simulink model "IEEE5BusSystemModel"  (R2017a)
settings: Solver=VariableStepAuto  StartTime=0.0  StopTime=1  MaxStep=1e-4  RelTol=1e-3  EnableMultiTasking=on
libraries: powerlib x45
settings Model: Creator=Rodney Tan  LastModifiedBy=HP
settings OptimizationCC: LifeSpan=inf
settings DebuggingCC: SFUnexpectedBacktrackingDiag=warning  SFNoUnconditionalDefaultTransitionDiag=warning  SFExecutionAtInitializationDiag=none
settings GRTTargetCC: TargetLangStandard=C89/C90 (ANSI)  GeneratePreprocessorConditionals=Disable all
settings ConfigComp: CovMetricSettings=dw  CovHtmlReporting=on  CovSaveCumulativeToWorkspaceVar=on  CovSaveSingleToWorkspaceVar=on  CovExternalEMLEnable=off

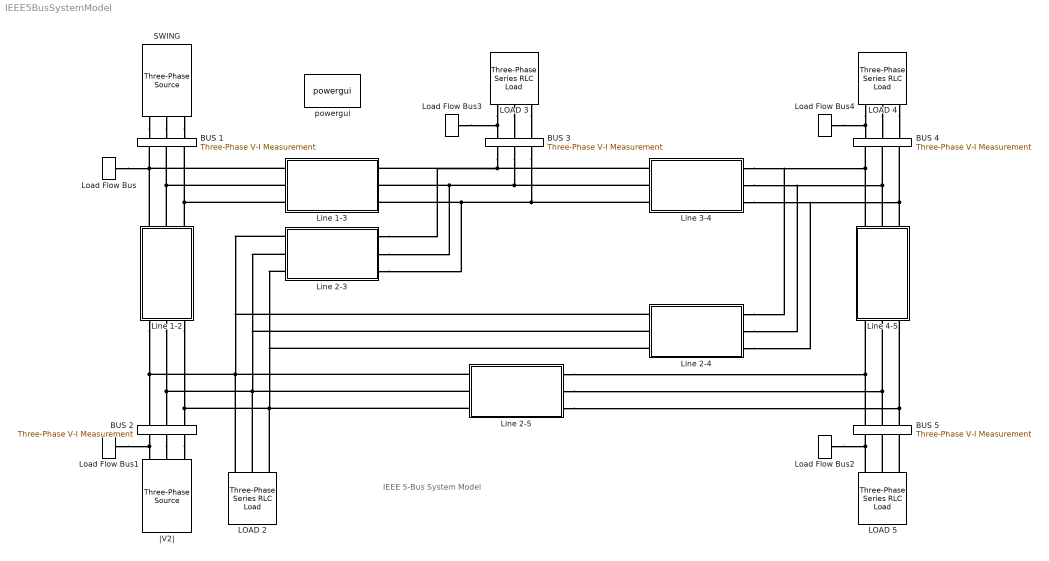
== system IEEE5BusSystemModel ==
  note: IEEE 5-Bus System Model
  BUS {1..5} (5 alike) : powerlib/Measurements/Three-Phase V-I Measurement  VoltageMeasurement=no  SetLabelV=off  LabelV=Vabc  Vpu=off  VpuLL=off  CurrentMeasurement=no  SetLabelI=off  LabelI=Iabc  Ipu=off  Pbase=100e6  Vbase=500e3  OutputType=Complex  PhasorSimulation=off  PSBequivalent=0
  LOAD 2 : powerlib/Elements/Three-Phase Series RLC Load  LConnTagsString=A|B|C  Configuration=Y (grounded)  NominalVoltage=10000  Vabc=[1e3 1e3 1e3]  Vabcp=[1e3 1e3 1e3]  NominalFrequency=60  UnbalancedPower=off  ActivePower=20e6  InductivePower=10e6  CapacitivePower=0  Pabc=[10e3 9e3 11e3]  QLabc=[100 90 110]  QCabc=[100 90 110]  Pabcp=[10e3 9e3 11e3]  QLabcp=[100 90 110]  QCabcp=[100 90 110]  Measurements=None  LoadType=constant PQ
  LOAD 3 : powerlib/Elements/Three-Phase Series RLC Load  LConnTagsString=A|B|C  Configuration=Y (grounded)  NominalVoltage=10000  Vabc=[1e3 1e3 1e3]  Vabcp=[1e3 1e3 1e3]  NominalFrequency=60  UnbalancedPower=off  ActivePower=45e6  InductivePower=15e6  CapacitivePower=0  Pabc=[10e3 9e3 11e3]  QLabc=[100 90 110]  QCabc=[100 90 110]  Pabcp=[10e3 9e3 11e3]  QLabcp=[100 90 110]  QCabcp=[100 90 110]  Measurements=None  LoadType=constant PQ
  LOAD 4 : powerlib/Elements/Three-Phase Series RLC Load  LConnTagsString=A|B|C  Configuration=Y (grounded)  NominalVoltage=(10000)  Vabc=[1e3 1e3 1e3]  Vabcp=[1e3 1e3 1e3]  NominalFrequency=60  UnbalancedPower=off  ActivePower=40e6  InductivePower=5e6  CapacitivePower=0  Pabc=[10e3 9e3 11e3]  QLabc=[100 90 110]  QCabc=[100 90 110]  Pabcp=[10e3 9e3 11e3]  QLabcp=[100 90 110]  QCabcp=[100 90 110]  Measurements=None  LoadType=constant PQ
  LOAD 5 : powerlib/Elements/Three-Phase Series RLC Load  LConnTagsString=A|B|C  Configuration=Y (grounded)  NominalVoltage=10000  Vabc=[1e3 1e3 1e3]  Vabcp=[1e3 1e3 1e3]  NominalFrequency=60  UnbalancedPower=off  ActivePower=60e6  InductivePower=10e6  CapacitivePower=0  Pabc=[10e3 9e3 11e3]  QLabc=[100 90 110]  QCabc=[100 90 110]  Pabcp=[10e3 9e3 11e3]  QLabcp=[100 90 110]  QCabcp=[100 90 110]  Measurements=None  LoadType=constant PQ
  Line 1-2 : Subsystem  mask{F=60, R=0.02, xL=0.06, B=0.03}
      mask prompts: F "Line Frequency (Hz)"; R "Line Resistance (pu)"; xL "Line Inductance (pu)"; B "Line Susceptance (pu)"
      mask Display:
      | disp('Line');
      | port_label('lconn',1,'A');
      | port_label('lconn',2,'B');
      | port_label('lconn',3,'C');
      | port_label('rconn',1,'a');
      | port_label('rconn',2,'b');
      | port_label('rconn',3,'c');
  Line 1-3 : Subsystem  mask{F=60, R=0.08, xL=0.24, B=0.025}
      mask prompts: F "Line Frequency (Hz)"; R "Line Resistance (pu)"; xL "Line Inductance (pu)"; B "Line Susceptance (pu)"
      mask Display:
      | disp('Line');
      | port_label('lconn',1,'A');
      | port_label('lconn',2,'B');
      | port_label('lconn',3,'C');
      | port_label('rconn',1,'a');
      | port_label('rconn',2,'b');
      | port_label('rconn',3,'c');
  Line 2-3 : Subsystem  mask{F=60, R=0.06, xL=0.18, B=0.02}
      mask prompts: F "Line Frequency (Hz)"; R "Line Resistance (pu)"; xL "Line Inductance (pu)"; B "Line Susceptance (pu)"
      mask Display:
      | disp('Line');
      | port_label('lconn',1,'A');
      | port_label('lconn',2,'B');
      | port_label('lconn',3,'C');
      | port_label('rconn',1,'a');
      | port_label('rconn',2,'b');
      | port_label('rconn',3,'c');
  Line 2-4 : Subsystem  mask{F=60, R=0.06, xL=0.18, B=0.02}
      mask prompts: F "Line Frequency (Hz)"; R "Line Resistance (pu)"; xL "Line Inductance (pu)"; B "Line Susceptance (pu)"
      mask Display:
      | disp('Line');
      | port_label('lconn',1,'A');
      | port_label('lconn',2,'B');
      | port_label('lconn',3,'C');
      | port_label('rconn',1,'a');
      | port_label('rconn',2,'b');
      | port_label('rconn',3,'c');
  Line 2-5 : Subsystem  mask{F=60, R=0.04, xL=0.12, B=0.015}
      mask prompts: F "Line Frequency (Hz)"; R "Line Resistance (pu)"; xL "Line Inductance (pu)"; B "Line Susceptance (pu)"
      mask Display:
      | disp('Line');
      | port_label('lconn',1,'A');
      | port_label('lconn',2,'B');
      | port_label('lconn',3,'C');
      | port_label('rconn',1,'a');
      | port_label('rconn',2,'b');
      | port_label('rconn',3,'c');
  Line 3-4 : Subsystem  mask{F=60, R=0.01, xL=0.03, B=0.01}
      mask prompts: F "Line Frequency (Hz)"; R "Line Resistance (pu)"; xL "Line Inductance (pu)"; B "Line Susceptance (pu)"
      mask Display:
      | disp('Line');
      | port_label('lconn',1,'A');
      | port_label('lconn',2,'B');
      | port_label('lconn',3,'C');
      | port_label('rconn',1,'a');
      | port_label('rconn',2,'b');
      | port_label('rconn',3,'c');
  Line 4-5 : Subsystem  mask{F=60, R=0.08, xL=0.24, B=0.025}
      mask prompts: F "Line Frequency (Hz)"; R "Line Resistance (pu)"; xL "Line Inductance (pu)"; B "Line Susceptance (pu)"
      mask Display:
      | disp('Line');
      | port_label('lconn',1,'A');
      | port_label('lconn',2,'B');
      | port_label('lconn',3,'C');
      | port_label('rconn',1,'a');
      | port_label('rconn',2,'b');
      | port_label('rconn',3,'c');
  Load Flow Bus : powerlib/Measurements/Load Flow Bus  LConnTagsString=a  Phases=single  Connectors=on one side  ID=BUS_1  Vbase=10e3  Vref=1.06  Vangle=0  VLF=1.06  VLFb=1  VLFc=1  angleLF=0  angleLFb=0  angleLFc=0
      settings: SourceProductName=Simscape Power Systems
  Load Flow Bus1 : powerlib/Measurements/Load Flow Bus  LConnTagsString=a  Phases=single  Connectors=on one side  ID=BUS_2  Vbase=10e3  Vref=1  Vangle=0  VLF=1.047  VLFb=1  VLFc=1  angleLF=-2.806  angleLFb=0  angleLFc=0
      settings: SourceProductName=Simscape Power Systems
  Load Flow Bus2 : powerlib/Measurements/Load Flow Bus  LConnTagsString=a  Phases=single  Connectors=on one side  ID=BUS_5  Vbase=10e3  Vref=1  Vangle=0  VLF=1.018  VLFb=1  VLFc=1  angleLF=-6.15  angleLFb=0  angleLFc=0
      settings: SourceProductName=Simscape Power Systems
  Load Flow Bus3 : powerlib/Measurements/Load Flow Bus  LConnTagsString=a  Phases=single  Connectors=on one side  ID=BUS_3  Vbase=10e3  Vref=1  Vangle=0  VLF=1.024  VLFb=1  VLFc=1  angleLF=-4.997  angleLFb=0  angleLFc=0
      settings: SourceProductName=Simscape Power Systems
  Load Flow Bus4 : powerlib/Measurements/Load Flow Bus  LConnTagsString=a  Phases=single  Connectors=on one side  ID=BUS_4  Vbase=10e3  Vref=1  Vangle=0  VLF=1.024  VLFb=1  VLFc=1  angleLF=-5.329  angleLFb=0  angleLFc=0
      settings: SourceProductName=Simscape Power Systems
  SWING : powerlib/Electrical Sources/Three-Phase Source  InternalConnection=Yg  VoltagePhases=off  Voltage=(10000)*1.06  PhaseAngle=0  Voltage_phases=[25e3 25e3 25e3]/sqrt(3)  PhaseAngles_phases=[0 -120 +120]  Frequency=60  NonIdealSource=off  SpecifyImpedance=off  Resistance=0.8929  Inductance=16.58e-3  ShortCircuitLevel=100e6  BaseVoltage=25e3  XRratio=7  BusType=swing  Pref=10e3  Qref=0  Prefabc=[10e3, 10e3, 10e3]  Qrefabc=[0, 0, 0]  Qmin=0  Qmax=0
  powergui : powerlib/powergui  Priority=1  SimulationMode=Continuous  SampleTime=50e-6  frequency=60  Iterations=50  frequencyindice=60  Pbase=100e6  ErrMax=0.0001  UnitsV=kV  UnitsW=MW  buscounter=0  FunctionMessages=off  echomessages=off  EnableUseOfTLC=off  CurrentSourceSwitches=off  DisableSnubberDevices=off  DisableRonSwitches=off  DisableVfSwitches=off  DisplayEquations=off  SolverType=Tustin/Backward Euler (TBE)  Interpol=off  ExternalGateDelay=off  methode=off  Ts=100  x0status=blocks  SPID=on  SwTol=0  HookPort=off  RestoreLinks=warning  ResistiveCurrentMeasurement=off  Frange=[0:2:500]  Ylog=off  Xlog=on  ShowGrid=off  save=off  variable=ZData  structure=0  ZoomFFT=off  StartTime=0.0  cycles=1  DisplayStyle=1  fundamental=60  FreqAxis=off  MaxFrequency=1000  frequencyindicesteady=1  RmsSteady=1  display=off
  |V2| : powerlib/Electrical Sources/Three-Phase Source  InternalConnection=Yg  VoltagePhases=off  Voltage=10000  PhaseAngle=0  Voltage_phases=[25e3 25e3 25e3]/sqrt(3)  PhaseAngles_phases=[0 -120 +120]  Frequency=60  NonIdealSource=off  SpecifyImpedance=off  Resistance=0.8929  Inductance=16.58e-3  ShortCircuitLevel=100e6  BaseVoltage=25e3  XRratio=7  BusType=PV  Pref=40e6  Qref=30e6  Prefabc=[10e3, 10e3, 10e3]  Qrefabc=[0, 0, 0]  Qmin=30e6  Qmax=30e6
  connections:
  SWING/RConn2 -- BUS 1/LConn2
  SWING/RConn1 -- BUS 1/LConn1
  SWING/RConn3 -- BUS 1/LConn3
  Line 1-2/RConn1 -- BUS 1/RConn1 -- Load Flow Bus/LConn1 -- Line 1-3/LConn1
  Line 1-2/RConn2 -- Line 1-3/LConn2 -- BUS 1/RConn2
  Line 1-2/RConn3 -- Line 1-3/LConn3 -- BUS 1/RConn3
  Line 3-4/LConn1 -- Line 1-3/RConn1 -- Line 2-3/RConn1 -- BUS 3/RConn1
  Line 3-4/LConn2 -- BUS 3/RConn2 -- Line 2-3/RConn2 -- Line 1-3/RConn2
  Line 3-4/LConn3 -- BUS 3/RConn3 -- Line 2-3/RConn3 -- Line 1-3/RConn3
  Line 1-2/LConn1 -- BUS 2/LConn1 -- Line 2-5/LConn1 -- Line 2-4/LConn1 -- Line 2-3/LConn1 -- LOAD 2/LConn1
  Line 1-2/LConn2 -- LOAD 2/LConn2 -- Line 2-3/LConn2 -- Line 2-4/LConn2 -- Line 2-5/LConn2 -- BUS 2/LConn2
  Line 1-2/LConn3 -- Line 2-3/LConn3 -- Line 2-4/LConn3 -- LOAD 2/LConn3 -- Line 2-5/LConn3 -- BUS 2/LConn3
  BUS 2/RConn2 -- |V2|/RConn2
  BUS 2/RConn1 -- Load Flow Bus1/LConn1 -- |V2|/RConn1
  BUS 2/RConn3 -- |V2|/RConn3
  BUS 5/LConn1 -- Line 2-5/RConn1 -- Line 4-5/LConn1
  BUS 5/LConn2 -- Line 2-5/RConn2 -- Line 4-5/LConn2
  BUS 5/LConn3 -- Line 2-5/RConn3 -- Line 4-5/LConn3
  Line 4-5/RConn2 -- Line 2-4/RConn2 -- Line 3-4/RConn2 -- BUS 4/RConn2
  Line 4-5/RConn1 -- Line 2-4/RConn1 -- Line 3-4/RConn1 -- BUS 4/RConn1
  Line 4-5/RConn3 -- Line 2-4/RConn3 -- Line 3-4/RConn3 -- BUS 4/RConn3
  LOAD 5/LConn2 -- BUS 5/RConn2
  LOAD 5/LConn1 -- Load Flow Bus2/LConn1 -- BUS 5/RConn1
  LOAD 5/LConn3 -- BUS 5/RConn3
  LOAD 3/LConn1 -- Load Flow Bus3/LConn1 -- BUS 3/LConn1
  LOAD 3/LConn2 -- BUS 3/LConn2
  LOAD 3/LConn3 -- BUS 3/LConn3
  LOAD 4/LConn1 -- Load Flow Bus4/LConn1 -- BUS 4/LConn1
  LOAD 4/LConn2 -- BUS 4/LConn2
  LOAD 4/LConn3 -- BUS 4/LConn3

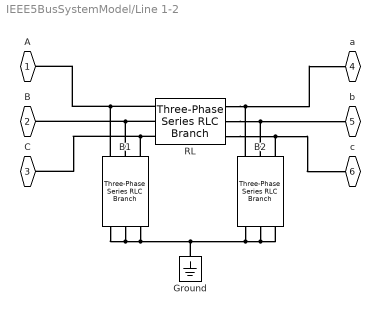
== system IEEE5BusSystemModel/Line 1-2 ==
  B1 : powerlib/Elements/Three-Phase Series RLC Branch  LConnTagsString=A|B|C  RConnTagsString=A|B|C  BranchType=C  Resistance=1e-6  Inductance=1e-3  Capacitance=B/(2*pi*F)  Measurements=None
  B2 : powerlib/Elements/Three-Phase Series RLC Branch  LConnTagsString=A|B|C  RConnTagsString=A|B|C  BranchType=C  Resistance=1e-6  Inductance=1e-3  Capacitance=B/(2*pi*F)  Measurements=None
  Ground : powerlib/Elements/Ground  LConnTagsString=a
  RL : powerlib/Elements/Three-Phase Series RLC Branch  LConnTagsString=A|B|C  RConnTagsString=A|B|C  BranchType=RL  Resistance=R  Inductance=xL/(2*pi*F)  Capacitance=1e-6  Measurements=None
  A : PMIOPort  Port=1  Side=Left
  B : PMIOPort  Port=2  Side=Left
  C : PMIOPort  Port=3  Side=Left
  a : PMIOPort  Port=4  Side=Right
  b : PMIOPort  Port=5  Side=Right
  c : PMIOPort  Port=6  Side=Right
  connections:
  RL/LConn1 -- A/RConn1 -- B1/LConn1
  RL/RConn1 -- a/RConn1 -- B2/LConn1
  RL/LConn2 -- B/RConn1 -- B1/LConn2
  RL/RConn2 -- b/RConn1 -- B2/LConn2
  RL/RConn3 -- B2/LConn3 -- c/RConn1
  RL/LConn3 -- B1/LConn3 -- C/RConn1
  B1/RConn1 -- B1/RConn2 -- B1/RConn3 -- B2/RConn1 -- B2/RConn2 -- B2/RConn3 -- Ground/LConn1

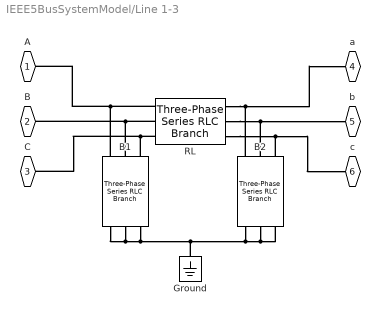
== system IEEE5BusSystemModel/Line 1-3 ==
  B1 : powerlib/Elements/Three-Phase Series RLC Branch  LConnTagsString=A|B|C  RConnTagsString=A|B|C  BranchType=C  Resistance=0  Inductance=1e-3  Capacitance=B/(2*pi*F)  Measurements=None
  B2 : powerlib/Elements/Three-Phase Series RLC Branch  LConnTagsString=A|B|C  RConnTagsString=A|B|C  BranchType=C  Resistance=1e-6  Inductance=1e-3  Capacitance=B/(2*pi*F)  Measurements=None
  Ground : powerlib/Elements/Ground  LConnTagsString=a
  RL : powerlib/Elements/Three-Phase Series RLC Branch  LConnTagsString=A|B|C  RConnTagsString=A|B|C  BranchType=RL  Resistance=R  Inductance=xL/(2*pi*F)  Capacitance=1e-6  Measurements=None
  A : PMIOPort  Port=1  Side=Left
  B : PMIOPort  Port=2  Side=Left
  C : PMIOPort  Port=3  Side=Left
  a : PMIOPort  Port=4  Side=Right
  b : PMIOPort  Port=5  Side=Right
  c : PMIOPort  Port=6  Side=Right
  connections:
  RL/LConn1 -- A/RConn1 -- B1/LConn1
  RL/RConn1 -- a/RConn1 -- B2/LConn1
  RL/LConn2 -- B/RConn1 -- B1/LConn2
  RL/RConn2 -- b/RConn1 -- B2/LConn2
  RL/RConn3 -- B2/LConn3 -- c/RConn1
  RL/LConn3 -- B1/LConn3 -- C/RConn1
  B1/RConn1 -- B1/RConn2 -- B1/RConn3 -- B2/RConn1 -- B2/RConn2 -- B2/RConn3 -- Ground/LConn1

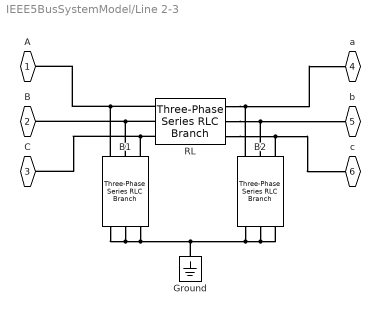
== system IEEE5BusSystemModel/Line 2-3 ==
  B1 : powerlib/Elements/Three-Phase Series RLC Branch  LConnTagsString=A|B|C  RConnTagsString=A|B|C  BranchType=C  Resistance=1e-6  Inductance=1e-3  Capacitance=B/(2*pi*F)  Measurements=None
  B2 : powerlib/Elements/Three-Phase Series RLC Branch  LConnTagsString=A|B|C  RConnTagsString=A|B|C  BranchType=C  Resistance=1e-6  Inductance=1e-3  Capacitance=B/(2*pi*F)  Measurements=None
  Ground : powerlib/Elements/Ground  LConnTagsString=a
  RL : powerlib/Elements/Three-Phase Series RLC Branch  LConnTagsString=A|B|C  RConnTagsString=A|B|C  BranchType=RL  Resistance=R  Inductance=xL/(2*pi*F)  Capacitance=1e-6  Measurements=None
  A : PMIOPort  Port=1  Side=Left
  B : PMIOPort  Port=2  Side=Left
  C : PMIOPort  Port=3  Side=Left
  a : PMIOPort  Port=4  Side=Right
  b : PMIOPort  Port=5  Side=Right
  c : PMIOPort  Port=6  Side=Right
  connections:
  RL/LConn1 -- A/RConn1 -- B1/LConn1
  RL/RConn1 -- a/RConn1 -- B2/LConn1
  RL/LConn2 -- B/RConn1 -- B1/LConn2
  RL/RConn2 -- b/RConn1 -- B2/LConn2
  RL/RConn3 -- B2/LConn3 -- c/RConn1
  RL/LConn3 -- B1/LConn3 -- C/RConn1
  B1/RConn1 -- B1/RConn2 -- B1/RConn3 -- B2/RConn1 -- B2/RConn2 -- B2/RConn3 -- Ground/LConn1

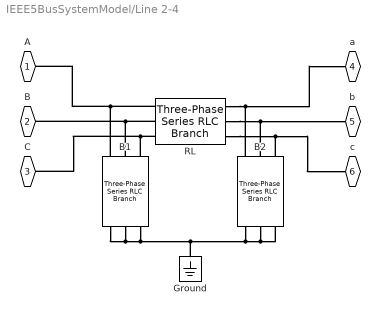
== system IEEE5BusSystemModel/Line 2-4 ==
  B1 : powerlib/Elements/Three-Phase Series RLC Branch  LConnTagsString=A|B|C  RConnTagsString=A|B|C  BranchType=C  Resistance=1e-6  Inductance=1e-3  Capacitance=B/(2*pi*F)  Measurements=None
  B2 : powerlib/Elements/Three-Phase Series RLC Branch  LConnTagsString=A|B|C  RConnTagsString=A|B|C  BranchType=C  Resistance=1e-6  Inductance=1e-3  Capacitance=B/(2*pi*F)  Measurements=None
  Ground : powerlib/Elements/Ground  LConnTagsString=a
  RL : powerlib/Elements/Three-Phase Series RLC Branch  LConnTagsString=A|B|C  RConnTagsString=A|B|C  BranchType=RL  Resistance=R  Inductance=xL/(2*pi*F)  Capacitance=1e-6  Measurements=None
  A : PMIOPort  Port=1  Side=Left
  B : PMIOPort  Port=2  Side=Left
  C : PMIOPort  Port=3  Side=Left
  a : PMIOPort  Port=4  Side=Right
  b : PMIOPort  Port=5  Side=Right
  c : PMIOPort  Port=6  Side=Right
  connections:
  RL/LConn1 -- A/RConn1 -- B1/LConn1
  RL/RConn1 -- a/RConn1 -- B2/LConn1
  RL/LConn2 -- B/RConn1 -- B1/LConn2
  RL/RConn2 -- b/RConn1 -- B2/LConn2
  RL/RConn3 -- B2/LConn3 -- c/RConn1
  RL/LConn3 -- B1/LConn3 -- C/RConn1
  B1/RConn1 -- B1/RConn2 -- B1/RConn3 -- B2/RConn1 -- B2/RConn2 -- B2/RConn3 -- Ground/LConn1

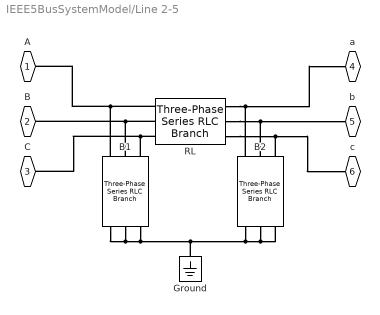
== system IEEE5BusSystemModel/Line 2-5 ==
  B1 : powerlib/Elements/Three-Phase Series RLC Branch  LConnTagsString=A|B|C  RConnTagsString=A|B|C  BranchType=C  Resistance=1e-6  Inductance=1e-3  Capacitance=B/(2*pi*F)  Measurements=None
  B2 : powerlib/Elements/Three-Phase Series RLC Branch  LConnTagsString=A|B|C  RConnTagsString=A|B|C  BranchType=C  Resistance=1e-6  Inductance=1e-3  Capacitance=B/(2*pi*F)  Measurements=None
  Ground : powerlib/Elements/Ground  LConnTagsString=a
  RL : powerlib/Elements/Three-Phase Series RLC Branch  LConnTagsString=A|B|C  RConnTagsString=A|B|C  BranchType=RL  Resistance=R  Inductance=xL/(2*pi*F)  Capacitance=1e-6  Measurements=None
  A : PMIOPort  Port=1  Side=Left
  B : PMIOPort  Port=2  Side=Left
  C : PMIOPort  Port=3  Side=Left
  a : PMIOPort  Port=4  Side=Right
  b : PMIOPort  Port=5  Side=Right
  c : PMIOPort  Port=6  Side=Right
  connections:
  RL/LConn1 -- A/RConn1 -- B1/LConn1
  RL/RConn1 -- a/RConn1 -- B2/LConn1
  RL/LConn2 -- B/RConn1 -- B1/LConn2
  RL/RConn2 -- b/RConn1 -- B2/LConn2
  RL/RConn3 -- B2/LConn3 -- c/RConn1
  RL/LConn3 -- B1/LConn3 -- C/RConn1
  B1/RConn1 -- B1/RConn2 -- B1/RConn3 -- B2/RConn1 -- B2/RConn2 -- B2/RConn3 -- Ground/LConn1

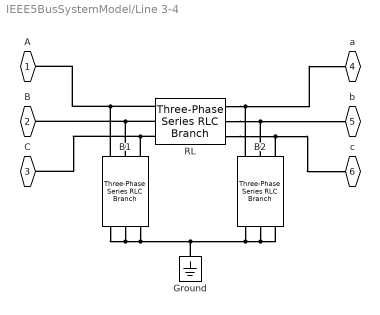
== system IEEE5BusSystemModel/Line 3-4 ==
  B1 : powerlib/Elements/Three-Phase Series RLC Branch  LConnTagsString=A|B|C  RConnTagsString=A|B|C  BranchType=C  Resistance=1e-6  Inductance=1e-3  Capacitance=B/(2*pi*F)  Measurements=None
  B2 : powerlib/Elements/Three-Phase Series RLC Branch  LConnTagsString=A|B|C  RConnTagsString=A|B|C  BranchType=C  Resistance=1e-6  Inductance=1e-3  Capacitance=B/(2*pi*F)  Measurements=None
  Ground : powerlib/Elements/Ground  LConnTagsString=a
  RL : powerlib/Elements/Three-Phase Series RLC Branch  LConnTagsString=A|B|C  RConnTagsString=A|B|C  BranchType=RL  Resistance=R  Inductance=xL/(2*pi*F)  Capacitance=1e-6  Measurements=None
  A : PMIOPort  Port=1  Side=Left
  B : PMIOPort  Port=2  Side=Left
  C : PMIOPort  Port=3  Side=Left
  a : PMIOPort  Port=4  Side=Right
  b : PMIOPort  Port=5  Side=Right
  c : PMIOPort  Port=6  Side=Right
  connections:
  RL/LConn1 -- A/RConn1 -- B1/LConn1
  RL/RConn1 -- a/RConn1 -- B2/LConn1
  RL/LConn2 -- B/RConn1 -- B1/LConn2
  RL/RConn2 -- b/RConn1 -- B2/LConn2
  RL/RConn3 -- B2/LConn3 -- c/RConn1
  RL/LConn3 -- B1/LConn3 -- C/RConn1
  B1/RConn1 -- B1/RConn2 -- B1/RConn3 -- B2/RConn1 -- B2/RConn2 -- B2/RConn3 -- Ground/LConn1

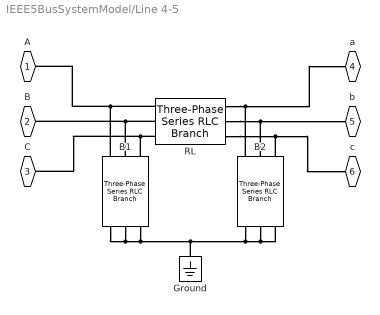
== system IEEE5BusSystemModel/Line 4-5 ==
  B1 : powerlib/Elements/Three-Phase Series RLC Branch  LConnTagsString=A|B|C  RConnTagsString=A|B|C  BranchType=C  Resistance=1e-6  Inductance=1e-3  Capacitance=B/(2*pi*F)  Measurements=None
  B2 : powerlib/Elements/Three-Phase Series RLC Branch  LConnTagsString=A|B|C  RConnTagsString=A|B|C  BranchType=C  Resistance=1e-6  Inductance=1e-3  Capacitance=B/(2*pi*F)  Measurements=None
  Ground : powerlib/Elements/Ground  LConnTagsString=a
  RL : powerlib/Elements/Three-Phase Series RLC Branch  LConnTagsString=A|B|C  RConnTagsString=A|B|C  BranchType=RL  Resistance=R  Inductance=xL/(2*pi*F)  Capacitance=1e-6  Measurements=None
  A : PMIOPort  Port=1  Side=Left
  B : PMIOPort  Port=2  Side=Left
  C : PMIOPort  Port=3  Side=Left
  a : PMIOPort  Port=4  Side=Right
  b : PMIOPort  Port=5  Side=Right
  c : PMIOPort  Port=6  Side=Right
  connections:
  RL/LConn1 -- A/RConn1 -- B1/LConn1
  RL/RConn1 -- a/RConn1 -- B2/LConn1
  RL/LConn2 -- B/RConn1 -- B1/LConn2
  RL/RConn2 -- b/RConn1 -- B2/LConn2
  RL/RConn3 -- B2/LConn3 -- c/RConn1
  RL/LConn3 -- B1/LConn3 -- C/RConn1
  B1/RConn1 -- B1/RConn2 -- B1/RConn3 -- B2/RConn1 -- B2/RConn2 -- B2/RConn3 -- Ground/LConn1
